simulink model "act1"  (R2020a)
settings: Solver=ode1  StartTime=0.0  StopTime=10.0  FixedStep=0.1  RelTol=1e-3
values from neighbouring files (symbols this model uses):
  a_1 = 1    [act1_script.m]    (also in act2_script.m; act3_script.m = 2)
  a_2 = 2    [act1_script.m]    (also in act2_script.m; act3_script.m = 1)
settings Model: Creator=Jorjolo  LastModifiedBy=Jorjolo

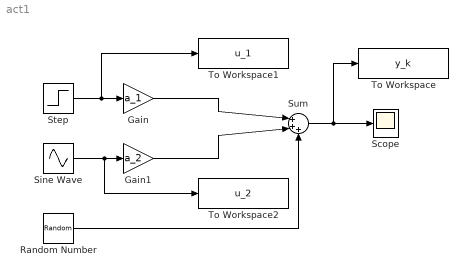
== system act1 ==
  Gain : Gain  Gain=a_1
  Gain1 : Gain  Gain=a_2
  Random Number : RandomNumber  Variance=0.1  SampleTime=0.1
  Scope : Scope
  Sine Wave : Sin  Frequency=10  Samples=100  SampleTime=0
  Step : Step  SampleTime=0
  Sum : Sum  Inputs=|+++
  To Workspace : ToWorkspace  VariableName=y_k  SampleTime=0.5
  To Workspace1 : ToWorkspace  VariableName=u_1  SampleTime=0.5
  To Workspace2 : ToWorkspace  VariableName=u_2  SampleTime=0.5
  wires:
  Sine Wave/1 -> To Workspace2/1, Gain1/1
  Step/1 -> To Workspace1/1, Gain/1
  Gain/1 -> Sum/1
  Gain1/1 -> Sum/2
  Sum/1 -> To Workspace/1, Scope/1
  Random Number/1 -> Sum/3
